simulink model "S_example4"  (Simulink 7.5)
settings: Solver=ode4  StartTime=0.0  StopTime=10.0  FixedStep=0.001  RelTol=1e-3
values from neighbouring files (symbols this model uses):
  N = 3.5    [S_example_4.m]
undefined symbols (not defined in the file or in its folder): Intercept_cruise_fcn
settings Model: Creator=CT  LastModifiedBy=CT

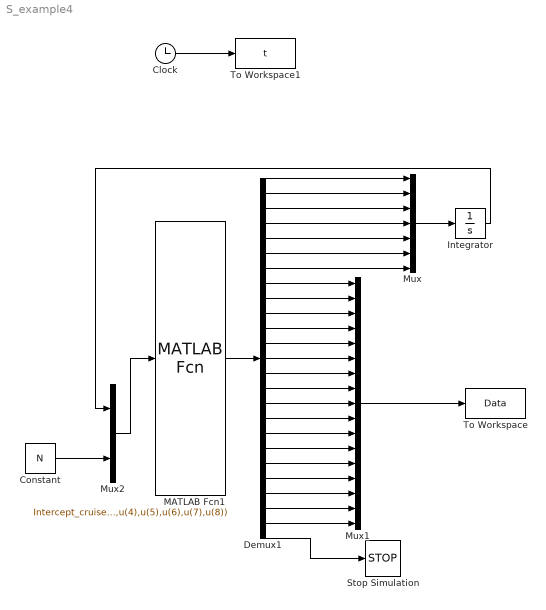
== system S_example4 ==
  Clock : Clock
      settings: Decimation=10
  Constant : Constant  Value=N  OutDataType=fixdt(1, 16)  OutScaling=2^0
  Demux1 : Demux  Outputs=25
  Integrator : Integrator  InitialCondition=[3000,2000,0,0,600,60*pi/180.0,-90*pi/180.0]
  MATLAB Fcn1 : MATLABFcn  MATLABFcn=Intercept_cruise_fcn(u(1),u(2),u(3),u(4),u(5),u(6),u(7),u(8))  OutputDimensions=25
  Mux : Mux  Inputs=7
  Mux1 : Mux  Inputs=17
  Mux2 : Mux  Inputs=2
  Stop Simulation : Stop
  To Workspace : ToWorkspace  VariableName=Data  SampleTime=-1  SaveFormat=Array
  To Workspace1 : ToWorkspace  VariableName=t  SampleTime=-1  SaveFormat=Array
  wires:
  MATLAB Fcn1/1 -> Demux1/1
  Demux1/1 -> Mux/1
  Demux1/2 -> Mux/2
  Demux1/3 -> Mux/3
  Demux1/4 -> Mux/4
  Demux1/5 -> Mux/5
  Demux1/6 -> Mux/6
  Mux/1 -> Integrator/1
  Demux1/7 -> Mux/7
  Demux1/8 -> Mux1/1
  Demux1/9 -> Mux1/2
  Demux1/10 -> Mux1/3
  Demux1/11 -> Mux1/4
  Demux1/12 -> Mux1/5
  Demux1/13 -> Mux1/6
  Demux1/14 -> Mux1/7
  Demux1/15 -> Mux1/8
  Demux1/16 -> Mux1/9
  Demux1/17 -> Mux1/10
  Demux1/18 -> Mux1/11
  Demux1/19 -> Mux1/12
  Demux1/20 -> Mux1/13
  Demux1/21 -> Mux1/14
  Demux1/22 -> Mux1/15
  Demux1/23 -> Mux1/16
  Demux1/24 -> Mux1/17
  Demux1/25 -> Stop Simulation/1
  Mux1/1 -> To Workspace/1
  Clock/1 -> To Workspace1/1
  Constant/1 -> Mux2/2
  Integrator/1 -> Mux2/1
  Mux2/1 -> MATLAB Fcn1/1
